simulink model "pnseq"  (R2019a)
settings: Solver=VariableStepAuto  StartTime=0.0  StopTime=10.0  RelTol=1e-3
settings Model: Creator=S&S LAB  LastModifiedBy=S&S LAB

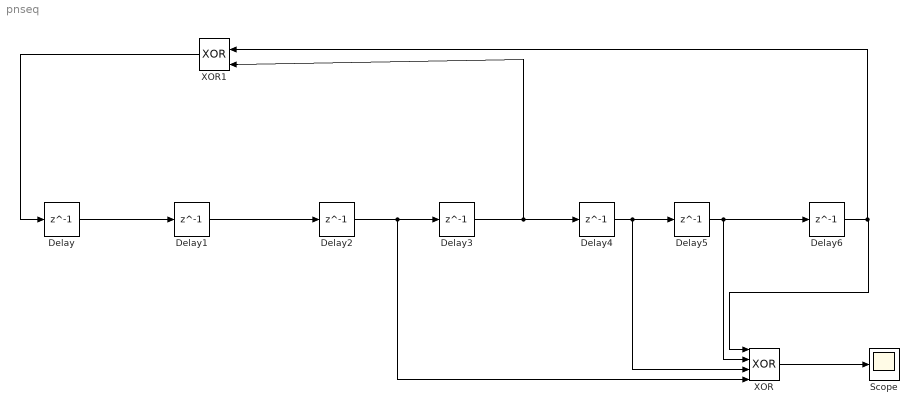
== system pnseq ==
  Delay{,1..6} (7 alike) : Delay  DelayLength=1  InitialCondition=0
  Scope : Scope
  XOR : Logic  Operator=XOR  Inputs=4  IconShape=distinctive  AllPortsSameDT=off  OutDataTypeStr=boolean
  XOR1 : Logic  Operator=XOR  IconShape=distinctive  AllPortsSameDT=off  OutDataTypeStr=boolean
  wires:
  Delay/1 -> Delay1/1
  Delay1/1 -> Delay2/1
  Delay2/1 -> XOR/4, Delay3/1
  Delay3/1 -> XOR1/2, Delay4/1
  Delay4/1 -> XOR/3, Delay5/1
  Delay5/1 -> XOR/2, Delay6/1
  Delay6/1 -> XOR1/1, XOR/1
  XOR1/1 -> Delay/1
  XOR/1 -> Scope/1
